simulink model "afe_abc_inv_psm_n"  (R2025b)
settings: Solver=ode1  StartTime=0.0  StopTime=simlength  FixedStep=tc  MaxStep=tc
values from neighbouring files (symbols this model uses):
  Adrso = eye(2) + Arso*ts_afe    [init_model.m]
  afe_pwm_phase_shift_mod1 = 0    [init_model.m]
  afe_pwm_phase_shift_mod2 = 0    [init_model.m]
  Aresd = eye(2) + Ares*ts_afe    [init_model.m]
  Bresd = Bres*ts_afe    [init_model.m]
  Cresd = Cres    [init_model.m]
  Crso = [1 0]    [init_model.m]
  CTRPIFF_CLIP_RELEASE = 0.001    [init_model.m]
  deepNEGeta = 0.5    [init_model.m]
  deepNEGxi = 0    [init_model.m]
  deepPOSxi = 0.5    [init_model.m]
  emf_fb_p = 0.2    [init_model.m]
  emf_fb_p_ccaller_1 = emf_fb_p    (= 0.2)    [init_model.m]
  emf_fb_p_ccaller_2 = emf_fb_p    (= 0.2)    [init_model.m]
  emf_p = emf_fb_p*4/10    (= 0.08)    [init_model.m]
  emf_p_ccaller_1 = emf_fb_p_ccaller_1*4/10    (= 0.08)    [init_model.m]
  emf_p_ccaller_2 = emf_fb_p_ccaller_2*4/10    (= 0.08)    [init_model.m]
  g0_161Hz = fcut_161Hz_flt * ts_afe * 2*pi    (= 0.126449104307)    [init_model.m]
  g0_1Hz = fcut_1Hz_flt * ts_afe * 2*pi    (= 0.000785398163397)    [init_model.m]
  g0_500Hz = fcut_500Hz_flt * ts_afe * 2*pi    (= 0.392699081699)    [init_model.m]
  g1_161Hz = 1 - g0_161Hz    (= 0.873550895693)    [init_model.m]
  g1_1Hz = 1 - g0_1Hz    (= 0.999214601837)    [init_model.m]
  g1_500Hz = 1 - g0_500Hz    (= 0.607300918301)    [init_model.m]
  i_grid_neg_eta_lim = 0.5    [init_model.m]
  i_grid_neg_eta_red_lim = 0.1    [init_model.m]
  i_grid_neg_xi_lim = 0.5    [init_model.m]
  i_grid_neg_xi_red_lim = 0.1    [init_model.m]
  i_grid_pos_eta_lim = 1    [init_model.m]
  i_grid_pos_eta_red_lim = 0.1    [init_model.m]
  id_lim = 0.35    [init_model.m]
  ieta_neg_ref_lim = 0.5    [init_model.m]
  ieta_pos_ref_lim = 1.0    (= 1)    [init_model.m]
  Igrid_phase_normalization_factor = 250e3/Vphase2/3/0.9*sqrt(2)    [init_model.m]
  inv_pwm_phase_shift_mod1 = 0    [init_model.m]
  iq_lim = 1.4    [init_model.m]
  ixi_pos_ref_lim = 1.6    [init_model.m]
  k_frt_ref = 2    [init_model.m]
  kg = Kobs(1)    [init_model.m]
  ki_afe = 45    [init_model.m]
  ki_align = 0.1    [init_model.m]
  ki_i = 18    [init_model.m]
  ki_rc_neg_grid = ki_rc_grid    (= 35)    [init_model.m]
  ki_rc_pos_grid = ki_rc_grid    (= 35)    [init_model.m]
  ki_vs = 35    [init_model.m]
  ki_w = 18    [init_model.m]
  kp_afe = 0.25    [init_model.m]
  kp_align = 0.6    [init_model.m]
  kp_i = 0.25    [init_model.m]
  kp_rc_neg_grid = kp_rc_grid    (= 0.35)    [init_model.m]
  kp_rc_pos_grid = kp_rc_grid    (= 0.35)    [init_model.m]
  kp_vs = 0.85    [init_model.m]
  kp_w = 2.5    [init_model.m]
  kw = Kobs(2)    [init_model.m]
  l1 = Kd(2)    [init_model.m]
  l2 = Kd(1)    [init_model.m]
  Ldrso = acker(Adrso',Crso',polesdrso)'    [init_model.m]
  lim_down_align = -0.2    [init_model.m]
  lim_up_align = 0.2    [init_model.m]
  mavarage_filter_frequency_base_order = 2    [init_model.m]
  motorc_m_scale = 2/3*Vdc_bez/ubez    [init_model.m]
  n1 = rms_perios/f_grid/ts_afe    [init_model.m]
  n10 = rms_perios/f_grid/ts_afe    [init_model.m]
  number_of_modules = 2    [init_model.m]
  omega_m_sim = omega_m_bez    [init_model.m]
  pll_i1 = 80    [init_model.m]
  pll_i1_ddsrt = pll_i1/2    (= 40)    [init_model.m]
  pll_p = 1    [init_model.m]
  pll_p_ddsrt = pll_p/2    (= 0.5)    [init_model.m]
  pll_p_frt = 0.2    [init_model.m]
  settle_time = 0.15    [init_model.m]
  simlength = 2    [init_model.m]
  start_time_LVRT = 2.0    (= 2)    [init_model.m]
  tc = ts_afe/200    (= 6.25e-07)    [init_model.m]
  time_aux_power_supply_fault = 1e3    (= 1000)    [init_model.m]
  time_gain_afe_module_1 = 1.0    (= 1)    [init_model.m]
  time_gain_afe_module_2 = 1.0    (= 1)    [init_model.m]
  time_gain_inv_module_1 = 1.0    (= 1)    [init_model.m]
  time_gain_inv_module_2 = 1.0    (= 1)    [init_model.m]
  time_phase_fault = 1e3    (= 1000)    [init_model.m]
  time_start_motor_control = 0.035    [init_model.m]
  transmission_delay = 125e-6*2    (= 0.00025)    [init_model.m]
  ts_afe = 1/fPWM_AFE/2    (= 0.000125)    [init_model.m]
  ts_inv = 1/fPWM_INV/2    (= 0.000125)    [init_model.m]
  Vdc_norm_ref = Vdc_ref/Vdc_nom    [init_model.m]
  Vdc_ref = 1070    [init_model.m]
  Vgrid_phase_normalization_factor = Vphase2*sqrt(2)    [init_model.m]
undefined symbols (not defined in the file or in its folder): Amplitude_U, Amplitude_V, Amplitude_W, end_time_LVRT, ibez, La, Lb, Ld_norm, Lq_norm, Ls_norm, magnitude, omega_bez, omega_grid_emulator_nom, omega_grid_nom, omega_m_bez, Phase_shift, psi_bez, psi_m, psi_m_norm, rpm_base, rpm_bez, Rs, Rs_norm, t_ramp, tau_bez, torque_base, ubez, ugrid_factor, V_phase_normalization_factor, Vdc_bez, Vemu_ref_norm, vn_eta_pu, vn_xi_pu, vp_xi_pu
libraries: fl_lib x215, nesl_utility x107, moving_average_filter x20, cstblocks x20, moving_average_filter_cc x16, simulink x6, threephase_inductor_lib x4, three_phase_pwm_modulator x4, single_phase_transformer_lib x3, power_meter_iec x1, flexshaft_lib x1, psm x1
(part 4 of 15)

== system afe_abc_inv_psm_n/afe_abc_inv_psm_mod1/afe/switch_2 ==
  Diode : fl_lib/Electrical/Electrical Elements/Diode  Vf=Vgamma V  Ron=Ron Ohm  Goff=1e-8 1/Ohm  i_specify=off  i_priority=None  i=0 A  i_nominal_specify=off  i_nominal_value=1  i_nominal_unit=A  v_specify=off  v_priority=None  v=0 V  v_nominal_specify=off  v_nominal_value=1  v_nominal_unit=V
  Switch : fl_lib/Electrical/Electrical Elements/Switch  R_closed=Ron Ohm  G_open=1e-8 1/Ohm  Threshold=7.5  i_specify=off  i_priority=None  i=0 A  i_nominal_specify=off  i_nominal_value=1  i_nominal_unit=A  v_specify=off  v_priority=None  v=0 V  v_nominal_specify=off  v_nominal_value=1  v_nominal_unit=V
  snubber : fl_lib/Electrical/Electrical Elements/Capacitor  c=Csnubber F  r=Rsnubber Ohm  g=0 1/Ohm  i_specify=off  i_priority=None  i=0 A  i_nominal_specify=off  i_nominal_value=1  i_nominal_unit=A  v_specify=off  v_priority=None  v=0 V  v_nominal_specify=off  v_nominal_value=1  v_nominal_unit=V  vc_specify=off  vc_priority=High  vc=0 V  vc_nominal_specify=off  vc_nominal_value=1  vc_nominal_unit=V
  G : PMIOPort  Side=Left
  C : PMIOPort  Port=2  Side=Left
  E : PMIOPort  Port=3  Side=Right
  connections:
  Switch/RConn2 -- C/RConn1 -- snubber/LConn1 -- Diode/RConn1
  Switch/RConn1 -- G/RConn1
  Switch/LConn1 -- E/RConn1 -- snubber/RConn1 -- Diode/LConn1

== system afe_abc_inv_psm_n/afe_abc_inv_psm_mod1/afe/switch_3 ==
  Diode : fl_lib/Electrical/Electrical Elements/Diode  Vf=Vgamma V  Ron=Ron Ohm  Goff=1e-8 1/Ohm  i_specify=off  i_priority=None  i=0 A  i_nominal_specify=off  i_nominal_value=1  i_nominal_unit=A  v_specify=off  v_priority=None  v=0 V  v_nominal_specify=off  v_nominal_value=1  v_nominal_unit=V
  Switch : fl_lib/Electrical/Electrical Elements/Switch  R_closed=Ron Ohm  G_open=1e-8 1/Ohm  Threshold=7.5  i_specify=off  i_priority=None  i=0 A  i_nominal_specify=off  i_nominal_value=1  i_nominal_unit=A  v_specify=off  v_priority=None  v=0 V  v_nominal_specify=off  v_nominal_value=1  v_nominal_unit=V
  snubber : fl_lib/Electrical/Electrical Elements/Capacitor  c=Csnubber F  r=Rsnubber Ohm  g=0 1/Ohm  i_specify=off  i_priority=None  i=0 A  i_nominal_specify=off  i_nominal_value=1  i_nominal_unit=A  v_specify=off  v_priority=None  v=0 V  v_nominal_specify=off  v_nominal_value=1  v_nominal_unit=V  vc_specify=off  vc_priority=High  vc=0 V  vc_nominal_specify=off  vc_nominal_value=1  vc_nominal_unit=V
  G : PMIOPort  Side=Left
  C : PMIOPort  Port=2  Side=Left
  E : PMIOPort  Port=3  Side=Right
  connections:
  Switch/RConn2 -- C/RConn1 -- snubber/LConn1 -- Diode/RConn1
  Switch/RConn1 -- G/RConn1
  Switch/LConn1 -- E/RConn1 -- snubber/RConn1 -- Diode/LConn1

== system afe_abc_inv_psm_n/afe_abc_inv_psm_mod1/afe/switch_4 ==
  Diode : fl_lib/Electrical/Electrical Elements/Diode  Vf=Vgamma V  Ron=Ron Ohm  Goff=1e-8 1/Ohm  i_specify=off  i_priority=None  i=0 A  i_nominal_specify=off  i_nominal_value=1  i_nominal_unit=A  v_specify=off  v_priority=None  v=0 V  v_nominal_specify=off  v_nominal_value=1  v_nominal_unit=V
  Switch : fl_lib/Electrical/Electrical Elements/Switch  R_closed=Ron Ohm  G_open=1e-8 1/Ohm  Threshold=7.5  i_specify=off  i_priority=None  i=0 A  i_nominal_specify=off  i_nominal_value=1  i_nominal_unit=A  v_specify=off  v_priority=None  v=0 V  v_nominal_specify=off  v_nominal_value=1  v_nominal_unit=V
  snubber : fl_lib/Electrical/Electrical Elements/Capacitor  c=Csnubber F  r=Rsnubber Ohm  g=0 1/Ohm  i_specify=off  i_priority=None  i=0 A  i_nominal_specify=off  i_nominal_value=1  i_nominal_unit=A  v_specify=off  v_priority=None  v=0 V  v_nominal_specify=off  v_nominal_value=1  v_nominal_unit=V  vc_specify=off  vc_priority=High  vc=0 V  vc_nominal_specify=off  vc_nominal_value=1  vc_nominal_unit=V
  G : PMIOPort  Side=Left
  C : PMIOPort  Port=2  Side=Left
  E : PMIOPort  Port=3  Side=Right
  connections:
  E/RConn1 -- Switch/LConn1 -- snubber/RConn1 -- Diode/LConn1
  Switch/RConn1 -- G/RConn1
  C/RConn1 -- Switch/RConn2 -- snubber/LConn1 -- Diode/RConn1

== system afe_abc_inv_psm_n/afe_abc_inv_psm_mod1/afe/switch_5 ==
  Diode : fl_lib/Electrical/Electrical Elements/Diode  Vf=Vgamma V  Ron=Ron Ohm  Goff=1e-8 1/Ohm  i_specify=off  i_priority=None  i=0 A  i_nominal_specify=off  i_nominal_value=1  i_nominal_unit=A  v_specify=off  v_priority=None  v=0 V  v_nominal_specify=off  v_nominal_value=1  v_nominal_unit=V
  Switch : fl_lib/Electrical/Electrical Elements/Switch  R_closed=Ron Ohm  G_open=1e-8 1/Ohm  Threshold=7.5  i_specify=off  i_priority=None  i=0 A  i_nominal_specify=off  i_nominal_value=1  i_nominal_unit=A  v_specify=off  v_priority=None  v=0 V  v_nominal_specify=off  v_nominal_value=1  v_nominal_unit=V
  snubber : fl_lib/Electrical/Electrical Elements/Capacitor  c=Csnubber F  r=Rsnubber Ohm  g=0 1/Ohm  i_specify=off  i_priority=None  i=0 A  i_nominal_specify=off  i_nominal_value=1  i_nominal_unit=A  v_specify=off  v_priority=None  v=0 V  v_nominal_specify=off  v_nominal_value=1  v_nominal_unit=V  vc_specify=off  vc_priority=High  vc=0 V  vc_nominal_specify=off  vc_nominal_value=1  vc_nominal_unit=V
  G : PMIOPort  Side=Left
  C : PMIOPort  Port=2  Side=Left
  E : PMIOPort  Port=3  Side=Right
  connections:
  Switch/RConn2 -- C/RConn1 -- snubber/LConn1 -- Diode/RConn1
  Switch/RConn1 -- G/RConn1
  Switch/LConn1 -- E/RConn1 -- snubber/RConn1 -- Diode/LConn1

== system afe_abc_inv_psm_n/afe_abc_inv_psm_mod1/afe/switch_6 ==
  Diode : fl_lib/Electrical/Electrical Elements/Diode  Vf=Vgamma V  Ron=Ron Ohm  Goff=1e-8 1/Ohm  i_specify=off  i_priority=None  i=0 A  i_nominal_specify=off  i_nominal_value=1  i_nominal_unit=A  v_specify=off  v_priority=None  v=0 V  v_nominal_specify=off  v_nominal_value=1  v_nominal_unit=V
  Switch : fl_lib/Electrical/Electrical Elements/Switch  R_closed=Ron Ohm  G_open=1e-8 1/Ohm  Threshold=7.5  i_specify=off  i_priority=None  i=0 A  i_nominal_specify=off  i_nominal_value=1  i_nominal_unit=A  v_specify=off  v_priority=None  v=0 V  v_nominal_specify=off  v_nominal_value=1  v_nominal_unit=V
  snubber : fl_lib/Electrical/Electrical Elements/Capacitor  c=Csnubber F  r=Rsnubber Ohm  g=0 1/Ohm  i_specify=off  i_priority=None  i=0 A  i_nominal_specify=off  i_nominal_value=1  i_nominal_unit=A  v_specify=off  v_priority=None  v=0 V  v_nominal_specify=off  v_nominal_value=1  v_nominal_unit=V  vc_specify=off  vc_priority=High  vc=0 V  vc_nominal_specify=off  vc_nominal_value=1  vc_nominal_unit=V
  G : PMIOPort  Side=Left
  C : PMIOPort  Port=2  Side=Left
  E : PMIOPort  Port=3  Side=Right
  connections:
  E/RConn1 -- Switch/LConn1 -- snubber/RConn1 -- Diode/LConn1
  Switch/RConn1 -- G/RConn1
  C/RConn1 -- Switch/RConn2 -- snubber/LConn1 -- Diode/RConn1

== system afe_abc_inv_psm_n/afe_abc_inv_psm_mod1/brake/switch_5 ==
  Diode : fl_lib/Electrical/Electrical Elements/Diode  Vf=Vgamma V  Ron=Ron Ohm  Goff=1e-8 1/Ohm  i_specify=off  i_priority=None  i=0 A  i_nominal_specify=off  i_nominal_value=1  i_nominal_unit=A  v_specify=off  v_priority=None  v=0 V  v_nominal_specify=off  v_nominal_value=1  v_nominal_unit=V
  Switch : fl_lib/Electrical/Electrical Elements/Switch  R_closed=Ron Ohm  G_open=1e-8 1/Ohm  Threshold=7.5  i_specify=off  i_priority=None  i=0 A  i_nominal_specify=off  i_nominal_value=1  i_nominal_unit=A  v_specify=off  v_priority=None  v=0 V  v_nominal_specify=off  v_nominal_value=1  v_nominal_unit=V
  G : PMIOPort  Side=Left
  C : PMIOPort  Port=2  Side=Left
  E : PMIOPort  Port=3  Side=Right
  connections:
  Switch/RConn2 -- C/RConn1 -- Diode/RConn1
  Switch/RConn1 -- G/RConn1
  Switch/LConn1 -- E/RConn1 -- Diode/LConn1

== system afe_abc_inv_psm_n/afe_abc_inv_psm_mod1/brake/switch_6 ==
  Diode : fl_lib/Electrical/Electrical Elements/Diode  Vf=Vgamma V  Ron=Ron Ohm  Goff=1e-8 1/Ohm  i_specify=off  i_priority=None  i=0 A  i_nominal_specify=off  i_nominal_value=1  i_nominal_unit=A  v_specify=off  v_priority=None  v=0 V  v_nominal_specify=off  v_nominal_value=1  v_nominal_unit=V
  C : PMIOPort  Side=Left
  E : PMIOPort  Port=2  Side=Right
  connections:
  E/RConn1 -- Diode/LConn1
  C/RConn1 -- Diode/RConn1

== system afe_abc_inv_psm_n/afe_abc_inv_psm_mod1/inverter/inverter ==
  duties_uvw : Inport
  Bus Selector : BusSelector  OutputSignals=gate_cmd_Q1,gate_cmd_Q2,gate_cmd_Q3,gate_cmd_Q4,gate_cmd_Q5,gate_cmd_Q6
  Current Sensor1 : fl_lib/Electrical/Electrical Sensors/Current Sensor
  Product{,1..5} (6 alike) : Product
  Simulink-PS Converter{,1..5} (6 alike) : nesl_utility/Simulink-PS Converter  PhysicalDomain=network_engine_domain  SubClassName=ps_input  LeftPortType=input  RightPortType=output  PseudoPeriodic=off  Frequencies=[]  NoiseDistribution=none  NoiseParameters=[]  Unit=1  AffineConversion=on  FilteringAndDerivatives=provide  SimscapeFilterOrder=1  InputFilterTimeConstant=0.001  UdotUserProvided=0
  Step : Step  Time=time_aux_power_supply_fault  Before=1  After=0  SampleTime=0
  ileg_dc_inv : nesl_utility/PS-Simulink Converter  PhysicalDomain=network_engine_domain  SubClassName=ps_output  LeftPortType=input  RightPortType=output  PseudoPeriodic=off  Frequencies=[]  VectorFormat=1-D array  Unit=A  AffineConversion=on
  sv_pwm : Subsystem
  switch_1 : Subsystem
      settings: PortSchema="{\"entries\":[{\"content\":{\"sides\":[{\"content\":{\"connectorIds\":[\"LConn1\"]},\"type\":\"ConnectorPlacement.EquallySpacedRectSide\",\"uuid\":\"9277da8d-d460-43e6-8478-dd662f15d226\"},{\"content\":{\"connectorIds\":[],\"side\":\"RIGHT\"},\"type\":\"ConnectorPlacement.EquallySpacedRectSide\",\"uuid\":\"a7ece396-f1d9-4f4f-a05b-db1fc65d6e1d\"},{\"content\":{\"connectorIds\":[\"LConn2\"],\"side\":\"TOP\"},\"type\":\"ConnectorPlacement.EquallySpacedRectSide\",\"uuid\":\"fdd70777-e9cf-4317-afb6-cae87f75d5b0\"},{\"content\":{\"connectorIds\":[\"RConn1\"],\"side\":\"BOTTOM\"},\"type\":\"ConnectorPlacement.EquallySpacedRectSide\",\"uuid\":\"2353ed68-b1a1-4775-9ca9-31e268d5443b\"}]},\"type\":\"ConnectorPlacement.EquallySpacedConnector\",\"uuid\":\"d5479f4c-4e65-4791-adcb-73df11f88590\"}],\"packageUris\":[\"http://schema.mathworks.com/mf0/Connector/R2020b\"],\"version\":\"1.0\"}"
  switch_2 : Subsystem
      settings: PortSchema="{\"entries\":[{\"content\":{\"sides\":[{\"content\":{\"connectorIds\":[\"LConn1\"]},\"type\":\"ConnectorPlacement.EquallySpacedRectSide\",\"uuid\":\"9277da8d-d460-43e6-8478-dd662f15d226\"},{\"content\":{\"connectorIds\":[],\"side\":\"RIGHT\"},\"type\":\"ConnectorPlacement.EquallySpacedRectSide\",\"uuid\":\"a7ece396-f1d9-4f4f-a05b-db1fc65d6e1d\"},{\"content\":{\"connectorIds\":[\"LConn2\"],\"side\":\"TOP\"},\"type\":\"ConnectorPlacement.EquallySpacedRectSide\",\"uuid\":\"fdd70777-e9cf-4317-afb6-cae87f75d5b0\"},{\"content\":{\"connectorIds\":[\"RConn1\"],\"side\":\"BOTTOM\"},\"type\":\"ConnectorPlacement.EquallySpacedRectSide\",\"uuid\":\"2353ed68-b1a1-4775-9ca9-31e268d5443b\"}]},\"type\":\"ConnectorPlacement.EquallySpacedConnector\",\"uuid\":\"d5479f4c-4e65-4791-adcb-73df11f88590\"}],\"packageUris\":[\"http://schema.mathworks.com/mf0/Connector/R2020b\"],\"version\":\"1.0\"}"
  switch_3 : Subsystem
      settings: PortSchema="{\"entries\":[{\"content\":{\"sides\":[{\"content\":{\"connectorIds\":[\"LConn1\"]},\"type\":\"ConnectorPlacement.EquallySpacedRectSide\",\"uuid\":\"9277da8d-d460-43e6-8478-dd662f15d226\"},{\"content\":{\"connectorIds\":[],\"side\":\"RIGHT\"},\"type\":\"ConnectorPlacement.EquallySpacedRectSide\",\"uuid\":\"a7ece396-f1d9-4f4f-a05b-db1fc65d6e1d\"},{\"content\":{\"connectorIds\":[\"LConn2\"],\"side\":\"TOP\"},\"type\":\"ConnectorPlacement.EquallySpacedRectSide\",\"uuid\":\"fdd70777-e9cf-4317-afb6-cae87f75d5b0\"},{\"content\":{\"connectorIds\":[\"RConn1\"],\"side\":\"BOTTOM\"},\"type\":\"ConnectorPlacement.EquallySpacedRectSide\",\"uuid\":\"2353ed68-b1a1-4775-9ca9-31e268d5443b\"}]},\"type\":\"ConnectorPlacement.EquallySpacedConnector\",\"uuid\":\"d5479f4c-4e65-4791-adcb-73df11f88590\"}],\"packageUris\":[\"http://schema.mathworks.com/mf0/Connector/R2020b\"],\"version\":\"1.0\"}"
  switch_4 : Subsystem
      settings: PortSchema="{\"entries\":[{\"content\":{\"sides\":[{\"content\":{\"connectorIds\":[\"LConn1\"]},\"type\":\"ConnectorPlacement.EquallySpacedRectSide\",\"uuid\":\"9277da8d-d460-43e6-8478-dd662f15d226\"},{\"content\":{\"connectorIds\":[],\"side\":\"RIGHT\"},\"type\":\"ConnectorPlacement.EquallySpacedRectSide\",\"uuid\":\"a7ece396-f1d9-4f4f-a05b-db1fc65d6e1d\"},{\"content\":{\"connectorIds\":[\"LConn2\"],\"side\":\"TOP\"},\"type\":\"ConnectorPlacement.EquallySpacedRectSide\",\"uuid\":\"fdd70777-e9cf-4317-afb6-cae87f75d5b0\"},{\"content\":{\"connectorIds\":[\"RConn1\"],\"side\":\"BOTTOM\"},\"type\":\"ConnectorPlacement.EquallySpacedRectSide\",\"uuid\":\"2353ed68-b1a1-4775-9ca9-31e268d5443b\"}]},\"type\":\"ConnectorPlacement.EquallySpacedConnector\",\"uuid\":\"d5479f4c-4e65-4791-adcb-73df11f88590\"}],\"packageUris\":[\"http://schema.mathworks.com/mf0/Connector/R2020b\"],\"version\":\"1.0\"}"
  switch_5 : Subsystem
      settings: PortSchema="{\"entries\":[{\"content\":{\"sides\":[{\"content\":{\"connectorIds\":[\"LConn1\"]},\"type\":\"ConnectorPlacement.EquallySpacedRectSide\",\"uuid\":\"9277da8d-d460-43e6-8478-dd662f15d226\"},{\"content\":{\"connectorIds\":[],\"side\":\"RIGHT\"},\"type\":\"ConnectorPlacement.EquallySpacedRectSide\",\"uuid\":\"a7ece396-f1d9-4f4f-a05b-db1fc65d6e1d\"},{\"content\":{\"connectorIds\":[\"LConn2\"],\"side\":\"TOP\"},\"type\":\"ConnectorPlacement.EquallySpacedRectSide\",\"uuid\":\"fdd70777-e9cf-4317-afb6-cae87f75d5b0\"},{\"content\":{\"connectorIds\":[\"RConn1\"],\"side\":\"BOTTOM\"},\"type\":\"ConnectorPlacement.EquallySpacedRectSide\",\"uuid\":\"2353ed68-b1a1-4775-9ca9-31e268d5443b\"}]},\"type\":\"ConnectorPlacement.EquallySpacedConnector\",\"uuid\":\"d5479f4c-4e65-4791-adcb-73df11f88590\"}],\"packageUris\":[\"http://schema.mathworks.com/mf0/Connector/R2020b\"],\"version\":\"1.0\"}"
  switch_6 : Subsystem
      settings: PortSchema="{\"entries\":[{\"content\":{\"sides\":[{\"content\":{\"connectorIds\":[\"LConn1\"]},\"type\":\"ConnectorPlacement.EquallySpacedRectSide\",\"uuid\":\"9277da8d-d460-43e6-8478-dd662f15d226\"},{\"content\":{\"connectorIds\":[],\"side\":\"RIGHT\"},\"type\":\"ConnectorPlacement.EquallySpacedRectSide\",\"uuid\":\"a7ece396-f1d9-4f4f-a05b-db1fc65d6e1d\"},{\"content\":{\"connectorIds\":[\"LConn2\"],\"side\":\"TOP\"},\"type\":\"ConnectorPlacement.EquallySpacedRectSide\",\"uuid\":\"fdd70777-e9cf-4317-afb6-cae87f75d5b0\"},{\"content\":{\"connectorIds\":[\"RConn1\"],\"side\":\"BOTTOM\"},\"type\":\"ConnectorPlacement.EquallySpacedRectSide\",\"uuid\":\"2353ed68-b1a1-4775-9ca9-31e268d5443b\"}]},\"type\":\"ConnectorPlacement.EquallySpacedConnector\",\"uuid\":\"d5479f4c-4e65-4791-adcb-73df11f88590\"}],\"packageUris\":[\"http://schema.mathworks.com/mf0/Connector/R2020b\"],\"version\":\"1.0\"}"
  u : PMIOPort  Side=Left
  v : PMIOPort  Port=2  Side=Left
  w : PMIOPort  Port=3  Side=Left
  V+ : PMIOPort  Port=4  Side=Right
  V- : PMIOPort  Port=5  Side=Right
  tag scope: ileg_dc_inv_mod1=global
  wires:
  [I1] -> Simulink-PS Converter/1
  [I2] -> Simulink-PS Converter1/1
  [I3] -> Simulink-PS Converter2/1
  [I4] -> Simulink-PS Converter3/1
  [I5] -> Simulink-PS Converter4/1
  [I6] -> Simulink-PS Converter5/1
  sv_pwm/1(gate_cmds) -> Bus Selector/1
  ileg_dc_inv/1 -> [ileg_dc_inv_mod1]
  Product/1 -> [I1]
  Product3/1 -> [I4]
  Product4/1 -> [I5]
  Product5/1 -> [I6]
  Product2/1 -> [I3]
  Product1/1 -> [I2]
  Step/1 -> Product5/1, Product4/1, Product3/1, Product2/1, Product/1, Product1/1
  Bus Selector/1 -> Product/2  "<gate_cmd_Q1>"
  Bus Selector/2 -> Product1/2  "<gate_cmd_Q2>"
  Bus Selector/3 -> Product2/2  "<gate_cmd_Q3>"
  Bus Selector/4 -> Product3/2  "<gate_cmd_Q4>"
  Bus Selector/5 -> Product4/2  "<gate_cmd_Q5>"
  Bus Selector/6 -> Product5/2  "<gate_cmd_Q6>"
  duties_uvw/1 -> sv_pwm/1(duties_uvw)
  connections:
  Current Sensor1/LConn1 -- V+/RConn1 -- switch_5/LConn2 -- switch_3/LConn2
  V-/RConn1 -- switch_2/RConn1 -- switch_6/RConn1 -- switch_4/RConn1
  switch_1/LConn1 -- Simulink-PS Converter/RConn1
  switch_2/LConn1 -- Simulink-PS Converter1/RConn1
  switch_3/LConn1 -- Simulink-PS Converter2/RConn1
  switch_4/LConn1 -- Simulink-PS Converter3/RConn1
  switch_5/LConn1 -- Simulink-PS Converter4/RConn1
  switch_6/LConn1 -- Simulink-PS Converter5/RConn1
  u/RConn1 -- switch_2/LConn2 -- switch_1/RConn1
  v/RConn1 -- switch_4/LConn2 -- switch_3/RConn1
  w/RConn1 -- switch_6/LConn2 -- switch_5/RConn1
  switch_1/LConn2 -- Current Sensor1/RConn2
  Current Sensor1/RConn1 -- ileg_dc_inv/LConn1

== system afe_abc_inv_psm_n/afe_abc_inv_psm_mod2/AFE_control/afe_control ==
  ug_abc_pu : Inport
  udc_pu : Inport  Port=2
  ig_abc_pu : Inport  Port=3
  is_abc_pu : Inport  Port=4
  local_time : Inport  Port=5
  master_time : Inport  Port=6
  Trigger : TriggerPort  VariantControl=(inherit)  PortDimensions=1
  Constant : Constant  Value=Vdc_norm_ref
  FRT-VDE4110 : Subsystem
  To Workspace4 : ToWorkspace  VariableName=t_ts_afe_sim_mod2  SampleTime=-1
      settings: MaxDataPoints=Ns_afe
  current_ctrl : Subsystem
  data_to_worspace_module_1 : Subsystem
  grid_current_sequences_and_reactive_pwr_ctrl : Subsystem
  grid_voltage_phase_lock_loops : Subsystem
  grid_voltage_sequences : Subsystem
  ig afe quantizzation and one step delay : Subsystem
  instantaneus_power : Subsystem
  interesting scopes : Subsystem
  is afe quantizzation and one step delay : Subsystem
  islanding_mode_detector : Subsystem
  phase_compensation_1 : Subsystem
  power-meter mod1 : Scope  NumInputPorts=2
      settings: ActiveDisplayYMinimum=-41.328407089198727  ActiveDisplayYMaximum=23.571293495272425  DataLoggingVariableName=ScopeData9
  space_vector : Subsystem
  udc_acquisition : Subsystem
  udc_ctrl : Subsystem
  ug afe quantizzation and one step delay : Subsystem
  duvw : Outport
  AFE2_local_time_corr : Outport  Port=2
  tag scope: igd_abc_pu_mod2=global, isd_abc_pu_mod2=global, udcd_pu_afe_mod2=global, ugd_abc_pu_mod2=global
  wires:
  [ug_beta_pu_mod2] -> islanding_mode_detector/3(beta)
  ig afe quantizzation and one step delay/1(igd_abc_pu) -> [igd_abc_pu_mod2]
  is afe quantizzation and one step delay/1(isd_abc_pu) -> [isd_abc_pu_mod2]
  ug afe quantizzation and one step delay/1(ugd_abc_pu) -> [ugd_abc_pu_mod2]
  [ug_alpha_pu_mod2] -> islanding_mode_detector/2(alpha)
  [gamma_grid_pll_mod2] -> islanding_mode_detector/1(gamma)
  [pwr_act_grid_mod2] -> power-meter mod1/1  "pwr_act_grid_mod1(kW)"
  [pwr_react_grid_mod2] -> power-meter mod1/2  "pwr_react_grid_mod1(kVAr)"
  udc_acquisition/1(udcd_pu) -> [udcd_pu_afe_mod2]
  udc_pu/1 -> udc_acquisition/1(udc_pu)
  [udcd_pu_afe_mod2] -> udc_ctrl/1(udc_pu)
  [isd_abc_pu_mod2] -> current_ctrl/2(is_abc_pu)
  [igd_abc_pu_mod2] -> grid_current_sequences_and_reactive_pwr_ctrl/1(ig_abc_pu)
  [ugd_abc_pu_mod2] -> grid_voltage_phase_lock_loops/1(ug_abc_pu)
  ig_abc_pu/1 -> ig afe quantizzation and one step delay/1(ig_abc_pu)
  is_abc_pu/1 -> is afe quantizzation and one step delay/1(is_abc_pu)
  space_vector/1(duvw) -> duvw/1
  current_ctrl/1(uab_out) -> space_vector/1(uab_out)
  ug_abc_pu/1 -> ug afe quantizzation and one step delay/1(ug_abc_pu)
  udc_ctrl/1(i_xi_ref) -> current_ctrl/1(i_xi_ref)  "i_xi_ref"
  Constant/1 -> udc_ctrl/2(udc_pu_ref)
  local_time/1 -> [local_time], To Workspace4/1
  [local_time] -> phase_compensation_1/1(local_time)
  phase_compensation_1/1(y) -> AFE2_local_time_corr/1
  master_time/1 -> phase_compensation_1/2(master_time)

== system afe_abc_inv_psm_n/afe_abc_inv_psm_mod2/INV_control/inverter_control ==
  is_uvw : Inport
  udc_pu : Inport  Port=2
  local_time : Inport  Port=3
  master_time : Inport  Port=4
  master_torque_ref : Inport  Port=5
  theta_elec_psm : Inport  Port=6
  Trigger : TriggerPort  VariantControl=(inherit)  PortDimensions=1
  Bus Creator : BusCreator  Inputs=2
  Mux2 : Mux  Inputs=3
  To Workspace1 : ToWorkspace  VariableName=t_ts_inv_sim_mod2  SampleTime=-1
      settings: MaxDataPoints=Ns_afe
  Variant Source : VariantSource  VariantControls={use_torque_curve == 1, use_speed_control == 1}
  current_ctrl : Subsystem
  encoder-sensorless-switch : Subsystem
  is inv quantizzation and one step delay : Subsystem
  measurements : Subsystem
  omega_pu : Subsystem
  omega_ref/omega_mod2 : Scope  NumInputPorts=3
      settings: ActiveDisplayYMinimum=-1.3333452178372498  ActiveDisplayYMaximum=1.261433879815884  DataLoggingVariableName=ScopeData3
  phase_compensation_1 : Subsystem
  space_vector : Subsystem
  torque_reference : Subsystem
  udc_acquisition : Subsystem
  duvw : Outport  VectorParamsAs1DForOutWhenUnconnected=off
  INV2_local_time_corr : Outport  Port=2
  tag scope: isd_uvw_inv_mod2=global, udcd_pu_inv_mod2=global
  wires:
  is inv quantizzation and one step delay/1(isd_abc_pu) -> [isd_uvw_inv_mod2]
  is_uvw/1 -> is inv quantizzation and one step delay/1(is_abc_pu)
  udc_pu/1 -> udc_acquisition/1(udc_pu)
  udc_acquisition/1(udcd_pu) -> [udcd_pu_inv_mod2]
  master_torque_ref/1 -> Variant Source/2, Bus Creator/2  "master_torque_ref"
  torque_reference/1(torque_ref) -> Variant Source/1  "iq_ref"
  omega_pu/1(abs(omega_pu)) -> torque_reference/1(rotor speed)
  omega_pu/2(omega_pu) -> Bus Creator/1  "omega_hat_pu"
  [u_mot_pu_mod2] -> Mux2/3  "u_mot_pu_mod2"
  Mux2/1 -> omega_ref/omega_mod2/3
  [uq_pu_mod2] -> Mux2/2  "uq_pu_mod2"
  [ud_pu_mod2] -> Mux2/1  "ud_pu_mod2"
  Variant Source/1 -> current_ctrl/1(torque_ref), omega_ref/omega_mod2/2  "torque reference"
  Bus Creator/1 -> omega_ref/omega_mod2/1  "x"
  local_time/1 -> To Workspace1/1, [local_time]
  phase_compensation_1/1(y) -> INV2_local_time_corr/1
  master_time/1 -> phase_compensation_1/2(master_time)
  [local_time] -> phase_compensation_1/1(local_time)
  current_ctrl/1(uab) -> space_vector/1(uab)
  space_vector/1(duvw) -> duvw/1
  theta_elec_psm/1 -> encoder-sensorless-switch/1(theta_elec_psm)

== system afe_abc_inv_psm_n/afe_abc_inv_psm_mod2/LCL_filter/threephase_vi_measures_stack ==
  Bus Creator : BusCreator  Inputs=6
  Current Sensor : fl_lib/Electrical/Electrical Sensors/Current Sensor
  Current Sensor1 : fl_lib/Electrical/Electrical Sensors/Current Sensor
  Current Sensor2 : fl_lib/Electrical/Electrical Sensors/Current Sensor
  Electrical Reference1 : fl_lib/Electrical/Electrical Elements/Electrical Reference
  Gain : Gain  Gain=1/3
  Gain1 : Gain  Gain=1/Vgrid_phase_normalization_factor
  Gain2 : Gain  Gain=1/Vgrid_phase_normalization_factor
  Gain3 : Gain  Gain=1/Vgrid_phase_normalization_factor
  Gain4 : Gain  Gain=1/Igrid_phase_normalization_factor
  Gain5 : Gain  Gain=1/Igrid_phase_normalization_factor
  Gain6 : Gain  Gain=1/Igrid_phase_normalization_factor
  Gain7 : Gain  Gain=Igrid_phase_normalization_factor
  Gain8 : Gain  Gain=Vgrid_phase_normalization_factor
  Gain9 : Gain  Gain=Igrid_phase_normalization_factor
  Selector : Selector  InputPortWidth=6  IndexOptions=Index vector (dialog)  Indices=[1 2 3]  OutputSizes=1
  Selector1 : Selector  InputPortWidth=6  IndexOptions=Index vector (dialog)  Indices=[4 5 6]  OutputSizes=1
  Sum : Sum  Inputs=+++
  Voltage Sensor : fl_lib/Electrical/Electrical Sensors/Voltage Sensor
  Voltage Sensor1 : fl_lib/Electrical/Electrical Sensors/Voltage Sensor
  Voltage Sensor2 : fl_lib/Electrical/Electrical Sensors/Voltage Sensor
  ia_afe : nesl_utility/PS-Simulink Converter  PhysicalDomain=network_engine_domain  SubClassName=ps_output  LeftPortType=input  RightPortType=output  PseudoPeriodic=off  Frequencies=[]  VectorFormat=1-D array  Unit=A  AffineConversion=off
  ib_afe : nesl_utility/PS-Simulink Converter  PhysicalDomain=network_engine_domain  SubClassName=ps_output  LeftPortType=input  RightPortType=output  PseudoPeriodic=off  Frequencies=[]  VectorFormat=1-D array  Unit=A  AffineConversion=off
  ic_afe : nesl_utility/PS-Simulink Converter  PhysicalDomain=network_engine_domain  SubClassName=ps_output  LeftPortType=input  RightPortType=output  PseudoPeriodic=off  Frequencies=[]  VectorFormat=1-D array  Unit=A  AffineConversion=off
  is_abc/us_abc _mod2 : Scope  NumInputPorts=3
      settings: SampleTime=tc  ActiveDisplayYMinimum=-383.27868862774517  ActiveDisplayYMaximum=384.39078927767747
  ua_afe : nesl_utility/PS-Simulink Converter  PhysicalDomain=network_engine_domain  SubClassName=ps_output  LeftPortType=input  RightPortType=output  PseudoPeriodic=off  Frequencies=[]  VectorFormat=1-D array  Unit=V  AffineConversion=off
  ub_afe : nesl_utility/PS-Simulink Converter  PhysicalDomain=network_engine_domain  SubClassName=ps_output  LeftPortType=input  RightPortType=output  PseudoPeriodic=off  Frequencies=[]  VectorFormat=1-D array  Unit=V  AffineConversion=off
  uc_afe : nesl_utility/PS-Simulink Converter  PhysicalDomain=network_engine_domain  SubClassName=ps_output  LeftPortType=input  RightPortType=output  PseudoPeriodic=off  Frequencies=[]  VectorFormat=1-D array  Unit=V  AffineConversion=off
  Ua : PMIOPort  Side=Left
  ua : PMIOPort  Port=2  Side=Right
  Ub : PMIOPort  Port=3  Side=Left
  ub : PMIOPort  Port=4  Side=Right
  Uc : PMIOPort  Port=5  Side=Left
  uc : PMIOPort  Port=6  Side=Right
  tag scope: is_abc_pu_mod2=global, iz_afe_pu_mod2=global, vs_abc_pu_mod2=global
  wires:
  Gain9/1 -> is_abc/us_abc _mod2/3  "iz_afe_mod2"
  Gain8/1 -> is_abc/us_abc _mod2/2  "vs_abc_mod2"
  Gain7/1 -> is_abc/us_abc _mod2/1  "is_abc_mod2"
  Gain5/1 -> Sum/3, Bus Creator/6  "ic_afe_pu"
  Gain4/1 -> Bus Creator/5, Sum/2  "ib_afe_pu"
  Gain6/1 -> Bus Creator/4, Sum/1  "ia_afe_pu"
  Gain3/1 -> Bus Creator/3  "uc_afe_pu"
  Gain2/1 -> Bus Creator/2  "ub_afe_pu"
  Gain1/1 -> Bus Creator/1  "ua_afe_pu"
  [iz_afe_pu_mod2] -> Gain9/1
  Gain/1 -> [iz_afe_pu_mod2]
  Sum/1 -> Gain/1
  [vs_abc_pu_mod2] -> Gain8/1
  [is_abc_pu_mod2] -> Gain7/1
  Selector1/1 -> [is_abc_pu_mod2]
  uc_afe/1 -> Gain3/1  "uc_afe"
  ub_afe/1 -> Gain2/1  "ub_afe"
  ua_afe/1 -> Gain1/1  "ua_afe"
  ic_afe/1 -> Gain5/1  "ic_afe"
  ia_afe/1 -> Gain6/1  "ia_afe"
  ib_afe/1 -> Gain4/1  "ib_afe"
  Selector/1 -> [vs_abc_pu_mod2]
  Bus Creator/1 -> Selector1/1, Selector/1  "vi_data"
  connections:
  Current Sensor2/RConn2 -- uc/RConn1
  ic_afe/LConn1 -- Current Sensor2/RConn1
  ia_afe/LConn1 -- Current Sensor/RConn1
  ib_afe/LConn1 -- Current Sensor1/RConn1
  Voltage Sensor2/RConn1 -- uc_afe/LConn1
  Current Sensor1/RConn2 -- ub/RConn1
  Voltage Sensor/LConn1 -- Ua/RConn1 -- Current Sensor/LConn1
  Current Sensor2/LConn1 -- Uc/RConn1 -- Voltage Sensor2/LConn1
  Voltage Sensor1/RConn1 -- ub_afe/LConn1
  Current Sensor/RConn2 -- ua/RConn1
  Voltage Sensor/RConn1 -- ua_afe/LConn1
  Voltage Sensor1/RConn2 -- Voltage Sensor2/RConn2 -- Voltage Sensor/RConn2 -- Electrical Reference1/LConn1
  Voltage Sensor1/LConn1 -- Ub/RConn1 -- Current Sensor1/LConn1

== system afe_abc_inv_psm_n/afe_abc_inv_psm_mod2/LCL_filter/threephase_vi_measures_stack1 ==
  Bus Creator : BusCreator  Inputs=6
  Current Sensor : fl_lib/Electrical/Electrical Sensors/Current Sensor
  Current Sensor1 : fl_lib/Electrical/Electrical Sensors/Current Sensor
  Current Sensor2 : fl_lib/Electrical/Electrical Sensors/Current Sensor
  Electrical Reference1 : fl_lib/Electrical/Electrical Elements/Electrical Reference
  Gain : Gain  Gain=1/Vgrid_phase_normalization_factor
  Gain1 : Gain  Gain=1/Vgrid_phase_normalization_factor
  Gain10 : Gain  Gain=1/Igrid_phase_normalization_factor
  Gain2 : Gain  Gain=1/Vgrid_phase_normalization_factor
  Gain6 : Gain  Gain=1/Igrid_phase_normalization_factor
  Gain9 : Gain  Gain=1/Igrid_phase_normalization_factor
  Selector : Selector  InputPortWidth=6  IndexOptions=Index vector (dialog)  Indices=[1 2 3]  OutputSizes=1
  Selector1 : Selector  InputPortWidth=6  IndexOptions=Index vector (dialog)  Indices=[4 5 6]  OutputSizes=1
  Voltage Sensor : fl_lib/Electrical/Electrical Sensors/Voltage Sensor
  Voltage Sensor1 : fl_lib/Electrical/Electrical Sensors/Voltage Sensor
  Voltage Sensor2 : fl_lib/Electrical/Electrical Sensors/Voltage Sensor
  ia_grid : nesl_utility/PS-Simulink Converter  PhysicalDomain=network_engine_domain  SubClassName=ps_output  LeftPortType=input  RightPortType=output  PseudoPeriodic=off  Frequencies=[]  VectorFormat=1-D array  Unit=A  AffineConversion=off
  ib_grid : nesl_utility/PS-Simulink Converter  PhysicalDomain=network_engine_domain  SubClassName=ps_output  LeftPortType=input  RightPortType=output  PseudoPeriodic=off  Frequencies=[]  VectorFormat=1-D array  Unit=A  AffineConversion=off
  ic_grid : nesl_utility/PS-Simulink Converter  PhysicalDomain=network_engine_domain  SubClassName=ps_output  LeftPortType=input  RightPortType=output  PseudoPeriodic=off  Frequencies=[]  VectorFormat=1-D array  Unit=A  AffineConversion=off
  ig_abc/ug_abc _mod2 : Scope  NumInputPorts=2
      settings: SampleTime=tc  ActiveDisplayYMinimum=-335.78711  ActiveDisplayYMaximum=237.87058
  ua_grid : nesl_utility/PS-Simulink Converter  PhysicalDomain=network_engine_domain  SubClassName=ps_output  LeftPortType=input  RightPortType=output  PseudoPeriodic=off  Frequencies=[]  VectorFormat=1-D array  Unit=V  AffineConversion=off
  ub_grid : nesl_utility/PS-Simulink Converter  PhysicalDomain=network_engine_domain  SubClassName=ps_output  LeftPortType=input  RightPortType=output  PseudoPeriodic=off  Frequencies=[]  VectorFormat=1-D array  Unit=V  AffineConversion=off
  uc_grid : nesl_utility/PS-Simulink Converter  PhysicalDomain=network_engine_domain  SubClassName=ps_output  LeftPortType=input  RightPortType=output  PseudoPeriodic=off  Frequencies=[]  VectorFormat=1-D array  Unit=V  AffineConversion=off
  Ua : PMIOPort  Side=Left
  ua : PMIOPort  Port=2  Side=Right
  Ub : PMIOPort  Port=3  Side=Left
  ub : PMIOPort  Port=4  Side=Right
  Uc : PMIOPort  Port=5  Side=Left
  uc : PMIOPort  Port=6  Side=Right
  tag scope: ig_abc_pu_mod2=global, ug_abc_pu_mod2=global
  wires:
  Gain10/1 -> Bus Creator/6  "ic_grid_pu"
  Gain9/1 -> Bus Creator/5  "ib_grid_pu"
  Gain6/1 -> Bus Creator/4  "ia_grid_pu"
  Gain2/1 -> Bus Creator/3  "uc_grid_pu"
  Gain1/1 -> Bus Creator/2  "ub_grid_pu"
  Gain/1 -> Bus Creator/1  "ua_grid_pu"
  Bus Creator/1 -> Selector1/1, Selector/1  "vi_data"
  Selector/1 -> [ug_abc_pu_mod2]
  ib_grid/1 -> Gain9/1
  ia_grid/1 -> Gain6/1
  ic_grid/1 -> Gain10/1
  ua_grid/1 -> Gain/1
  ub_grid/1 -> Gain1/1
  uc_grid/1 -> Gain2/1
  Selector1/1 -> [ig_abc_pu_mod2]
  [ig_abc_pu_mod2] -> ig_abc/ug_abc _mod2/1  "ig_abc_mod2"
  [ug_abc_pu_mod2] -> ig_abc/ug_abc _mod2/2  "ug_abc_mod2"
  connections:
  Current Sensor1/LConn1 -- Ub/RConn1 -- Voltage Sensor1/LConn1
  Electrical Reference1/LConn1 -- Voltage Sensor/RConn2 -- Voltage Sensor2/RConn2 -- Voltage Sensor1/RConn2
  Voltage Sensor/RConn1 -- ua_grid/LConn1
  Current Sensor/RConn2 -- ua/RConn1
  Voltage Sensor1/RConn1 -- ub_grid/LConn1
  Voltage Sensor2/LConn1 -- Uc/RConn1 -- Current Sensor2/LConn1
  Current Sensor/LConn1 -- Ua/RConn1 -- Voltage Sensor/LConn1
  Current Sensor1/RConn2 -- ub/RConn1
  Voltage Sensor2/RConn1 -- uc_grid/LConn1
  ib_grid/LConn1 -- Current Sensor1/RConn1
  ia_grid/LConn1 -- Current Sensor/RConn1
  ic_grid/LConn1 -- Current Sensor2/RConn1
  Current Sensor2/RConn2 -- uc/RConn1

== system afe_abc_inv_psm_n/afe_abc_inv_psm_mod2/L_filter/threephase_vi_measures_stack ==
  Bus Creator : BusCreator  Inputs=6
  Current Sensor : fl_lib/Electrical/Electrical Sensors/Current Sensor
  Current Sensor1 : fl_lib/Electrical/Electrical Sensors/Current Sensor
  Current Sensor2 : fl_lib/Electrical/Electrical Sensors/Current Sensor
  Electrical Reference1 : fl_lib/Electrical/Electrical Elements/Electrical Reference
  Gain : Gain  Gain=1/ibez
  Gain1 : Gain  Gain=1/ibez
  Gain2 : Gain  Gain=1/ibez
  Gain3 : Gain  Gain=1/ubez
  Gain4 : Gain  Gain=1/ubez
  Gain5 : Gain  Gain=1/ubez
  Selector : Selector  InputPortWidth=6  IndexOptions=Index vector (dialog)  Indices=[1 2 3]  OutputSizes=1
  Selector1 : Selector  InputPortWidth=6  IndexOptions=Index vector (dialog)  Indices=[4 5 6]  OutputSizes=1
  Voltage Sensor : fl_lib/Electrical/Electrical Sensors/Voltage Sensor
  Voltage Sensor1 : fl_lib/Electrical/Electrical Sensors/Voltage Sensor
  Voltage Sensor2 : fl_lib/Electrical/Electrical Sensors/Voltage Sensor
  iu_inv : nesl_utility/PS-Simulink Converter  PhysicalDomain=network_engine_domain  SubClassName=ps_output  LeftPortType=input  RightPortType=output  PseudoPeriodic=off  Frequencies=[]  VectorFormat=1-D array  Unit=A  AffineConversion=off
  iv_inv : nesl_utility/PS-Simulink Converter  PhysicalDomain=network_engine_domain  SubClassName=ps_output  LeftPortType=input  RightPortType=output  PseudoPeriodic=off  Frequencies=[]  VectorFormat=1-D array  Unit=A  AffineConversion=off
  iw_inv : nesl_utility/PS-Simulink Converter  PhysicalDomain=network_engine_domain  SubClassName=ps_output  LeftPortType=input  RightPortType=output  PseudoPeriodic=off  Frequencies=[]  VectorFormat=1-D array  Unit=A  AffineConversion=off
  uu_inv : nesl_utility/PS-Simulink Converter  PhysicalDomain=network_engine_domain  SubClassName=ps_output  LeftPortType=input  RightPortType=output  PseudoPeriodic=off  Frequencies=[]  VectorFormat=1-D array  Unit=V  AffineConversion=off
  uv_inv : nesl_utility/PS-Simulink Converter  PhysicalDomain=network_engine_domain  SubClassName=ps_output  LeftPortType=input  RightPortType=output  PseudoPeriodic=off  Frequencies=[]  VectorFormat=1-D array  Unit=V  AffineConversion=off
  uw_inv : nesl_utility/PS-Simulink Converter  PhysicalDomain=network_engine_domain  SubClassName=ps_output  LeftPortType=input  RightPortType=output  PseudoPeriodic=off  Frequencies=[]  VectorFormat=1-D array  Unit=V  AffineConversion=off
  Uu : PMIOPort  Side=Left
  uu : PMIOPort  Port=2  Side=Right
  Uv : PMIOPort  Port=3  Side=Left
  uv : PMIOPort  Port=4  Side=Right
  Uw : PMIOPort  Port=5  Side=Left
  uw : PMIOPort  Port=6  Side=Right
  tag scope: is_uvw_pu_mod2=global, us_uvw_pu_mod2=global
  wires:
  Gain5/1 -> Bus Creator/3  "uw_inv_pu"
  Gain4/1 -> Bus Creator/2  "uv_inv_pu"
  Gain3/1 -> Bus Creator/1  "uu_inv_pu"
  Gain2/1 -> Bus Creator/6  "iw_inv_pu"
  Gain1/1 -> Bus Creator/5  "iv_inv_pu"
  Gain/1 -> Bus Creator/4  "iu_inv_pu"
  Selector1/1 -> [is_uvw_pu_mod2]
  uw_inv/1 -> Gain5/1  "uw_inv"
  uv_inv/1 -> Gain4/1  "uv_inv"
  uu_inv/1 -> Gain3/1  "uu_inv"
  iw_inv/1 -> Gain2/1  "iw_inv"
  iu_inv/1 -> Gain/1  "iu_inv"
  iv_inv/1 -> Gain1/1  "iv_inv"
  Selector/1 -> [us_uvw_pu_mod2]
  Bus Creator/1 -> Selector1/1, Selector/1  "vi_data"
  connections:
  Current Sensor2/RConn2 -- uw/RConn1
  iw_inv/LConn1 -- Current Sensor2/RConn1
  iu_inv/LConn1 -- Current Sensor/RConn1
  iv_inv/LConn1 -- Current Sensor1/RConn1
  Voltage Sensor2/RConn1 -- uw_inv/LConn1
  Current Sensor1/RConn2 -- uv/RConn1
  Voltage Sensor/LConn1 -- Uu/RConn1 -- Current Sensor/LConn1
  Current Sensor2/LConn1 -- Uw/RConn1 -- Voltage Sensor2/LConn1
  Voltage Sensor1/RConn1 -- uv_inv/LConn1
  Current Sensor/RConn2 -- uu/RConn1
  Voltage Sensor/RConn1 -- uu_inv/LConn1
  Voltage Sensor1/RConn2 -- Voltage Sensor2/RConn2 -- Voltage Sensor/RConn2 -- Electrical Reference1/LConn1
  Voltage Sensor1/LConn1 -- Uv/RConn1 -- Current Sensor1/LConn1

== system afe_abc_inv_psm_n/afe_abc_inv_psm_mod2/afe/dclink_measure ==
  Controlled Voltage Source : fl_lib/Electrical/Electrical Sources/Controlled Voltage Source
  Current Sensor1 : fl_lib/Electrical/Electrical Sensors/Current Sensor
  Electrical Reference : fl_lib/Electrical/Electrical Elements/Electrical Reference
  Gain : Gain  Gain=107.4e3
  Gain1 : Gain  Gain=1/Vdc_bez
  R_derating : Subsystem  Commented=on
  Resistor : fl_lib/Electrical/Electrical Elements/Resistor  R=107.4 kOhm  i_specify=off  i_priority=None  i=0 A  i_nominal_specify=off  i_nominal_value=1  i_nominal_unit=A  v_specify=off  v_priority=None  v=0 V  v_nominal_specify=off  v_nominal_value=1  v_nominal_unit=V
  Saturation : Saturate  UpperLimit=inf  LowerLimit=1
  Simulink-PS Converter : nesl_utility/Simulink-PS Converter  PhysicalDomain=network_engine_domain  SubClassName=ps_input  LeftPortType=input  RightPortType=output  PseudoPeriodic=off  Frequencies=[]  NoiseDistribution=none  NoiseParameters=[]  Unit=Ohm  AffineConversion=off  FilteringAndDerivatives=provide  SimscapeFilterOrder=1  InputFilterTimeConstant=0.001  UdotUserProvided=0
  Variable Resistor : fl_lib/Electrical/Electrical Elements/Variable Resistor  Rmin=0 Ohm  thermalEnable=false  thermal_mass=1 J/K  i_specify=off  i_priority=None  i=0 A  i_nominal_specify=off  i_nominal_value=1  i_nominal_unit=A  v_specify=off  v_priority=None  v=0 V  v_nominal_specify=off  v_nominal_value=1  v_nominal_unit=V  T_specify=off  T_priority=None  T=300 K  T_nominal_specify=off  T_nominal_value=1  T_nominal_unit=K
  dclink_voltage_measure_comparison mod2 : Scope  NumInputPorts=3
      settings: SampleTime=tc  ActiveDisplayYMinimum=439.20035  ActiveDisplayYMaximum=1355.17542
  im_udc : nesl_utility/PS-Simulink Converter  PhysicalDomain=network_engine_domain  SubClassName=ps_output  LeftPortType=input  RightPortType=output  PseudoPeriodic=off  Frequencies=[]  VectorFormat=1-D array  Unit=A  AffineConversion=on
  udc : PMIOPort  Side=Left
  tag scope: vdc_pu_afe_mod2=global, vdc_pu_inv_mod2=global
  wires:
  Gain1/1 -> [vdc_pu_afe_mod2], dclink_voltage_measure_comparison mod2/2, [vdc_pu_inv_mod2]
  R_derating/1(DR) -> Simulink-PS Converter/1
  [udc_mod2] -> dclink_voltage_measure_comparison mod2/3  "real"
  im_udc/1 -> Gain/1
  Saturation/1 -> Gain1/1
  Gain/1 -> dclink_voltage_measure_comparison mod2/1, Saturation/1  "measure_si"
  connections:
  Controlled Voltage Source/LConn1 -- Resistor/LConn1
  Simulink-PS Converter/RConn1 -- Variable Resistor/LConn1
  Current Sensor1/LConn1 -- Variable Resistor/RConn1
  Controlled Voltage Source/RConn2 -- Electrical Reference/LConn1 -- Current Sensor1/RConn2
  Current Sensor1/RConn1 -- im_udc/LConn1
  Resistor/RConn1 -- Variable Resistor/LConn2
  udc/RConn1 -- Controlled Voltage Source/RConn1

== system afe_abc_inv_psm_n/afe_abc_inv_psm_mod2/afe/sv_pwm ==
  duties_uvw : Inport
  Bus Selector2 : BusSelector  OutputSignals=du(k),dv(k),dw(k)
  Constant1 : Constant  Value=afe_pwm_phase_shift_mod2
  modulator1 : Subsystem
  td2tc_1 : TransferFcn  Denominator=[tc 1]
  td2tc_2 : TransferFcn  Denominator=[tc 1]
  td2tc_3 : TransferFcn  Denominator=[tc 1]
  gate_cmds : Outport
  wires:
  td2tc_2/1 -> modulator1/2(v)  "dv(t)"
  td2tc_3/1 -> modulator1/3(w)  "dw(t)"
  td2tc_1/1 -> modulator1/1(u)  "du(t)"
  duties_uvw/1 -> Bus Selector2/1
  Bus Selector2/3 -> td2tc_3/1  "<dw(k)>"
  Bus Selector2/2 -> td2tc_2/1  "<dv(k)>"
  Bus Selector2/1 -> td2tc_1/1  "<du(k)>"
  Constant1/1 -> modulator1/4(phase)
  modulator1/1(gate_cmds) -> gate_cmds/1

== system afe_abc_inv_psm_n/afe_abc_inv_psm_mod2/afe/switch_1 ==
  Diode : fl_lib/Electrical/Electrical Elements/Diode  Vf=Vgamma V  Ron=Ron Ohm  Goff=1e-8 1/Ohm  i_specify=off  i_priority=None  i=0 A  i_nominal_specify=off  i_nominal_value=1  i_nominal_unit=A  v_specify=off  v_priority=None  v=0 V  v_nominal_specify=off  v_nominal_value=1  v_nominal_unit=V
  Switch : fl_lib/Electrical/Electrical Elements/Switch  R_closed=Ron Ohm  G_open=1e-8 1/Ohm  Threshold=7.5  i_specify=off  i_priority=None  i=0 A  i_nominal_specify=off  i_nominal_value=1  i_nominal_unit=A  v_specify=off  v_priority=None  v=0 V  v_nominal_specify=off  v_nominal_value=1  v_nominal_unit=V
  snubber : fl_lib/Electrical/Electrical Elements/Capacitor  c=Csnubber F  r=Rsnubber Ohm  g=0 1/Ohm  i_specify=off  i_priority=None  i=0 A  i_nominal_specify=off  i_nominal_value=1  i_nominal_unit=A  v_specify=off  v_priority=None  v=0 V  v_nominal_specify=off  v_nominal_value=1  v_nominal_unit=V  vc_specify=off  vc_priority=High  vc=0 V  vc_nominal_specify=off  vc_nominal_value=1  vc_nominal_unit=V
  G : PMIOPort  Side=Left
  C : PMIOPort  Port=2  Side=Left
  E : PMIOPort  Port=3  Side=Right
  connections:
  Switch/RConn2 -- C/RConn1 -- Diode/RConn1 -- snubber/LConn1
  Switch/RConn1 -- G/RConn1
  Switch/LConn1 -- E/RConn1 -- snubber/RConn1 -- Diode/LConn1

== system afe_abc_inv_psm_n/afe_abc_inv_psm_mod2/afe/switch_2 ==
  Diode : fl_lib/Electrical/Electrical Elements/Diode  Vf=Vgamma V  Ron=Ron Ohm  Goff=1e-8 1/Ohm  i_specify=off  i_priority=None  i=0 A  i_nominal_specify=off  i_nominal_value=1  i_nominal_unit=A  v_specify=off  v_priority=None  v=0 V  v_nominal_specify=off  v_nominal_value=1  v_nominal_unit=V
  Switch : fl_lib/Electrical/Electrical Elements/Switch  R_closed=Ron Ohm  G_open=1e-8 1/Ohm  Threshold=7.5  i_specify=off  i_priority=None  i=0 A  i_nominal_specify=off  i_nominal_value=1  i_nominal_unit=A  v_specify=off  v_priority=None  v=0 V  v_nominal_specify=off  v_nominal_value=1  v_nominal_unit=V
  snubber : fl_lib/Electrical/Electrical Elements/Capacitor  c=Csnubber F  r=Rsnubber Ohm  g=0 1/Ohm  i_specify=off  i_priority=None  i=0 A  i_nominal_specify=off  i_nominal_value=1  i_nominal_unit=A  v_specify=off  v_priority=None  v=0 V  v_nominal_specify=off  v_nominal_value=1  v_nominal_unit=V  vc_specify=off  vc_priority=High  vc=0 V  vc_nominal_specify=off  vc_nominal_value=1  vc_nominal_unit=V
  G : PMIOPort  Side=Left
  C : PMIOPort  Port=2  Side=Left
  E : PMIOPort  Port=3  Side=Right
  connections:
  Diode/LConn1 -- snubber/RConn1 -- E/RConn1 -- Switch/LConn1
  Switch/RConn1 -- G/RConn1
  Diode/RConn1 -- snubber/LConn1 -- C/RConn1 -- Switch/RConn2

== system afe_abc_inv_psm_n/afe_abc_inv_psm_mod2/afe/switch_3 ==
  Diode : fl_lib/Electrical/Electrical Elements/Diode  Vf=Vgamma V  Ron=Ron Ohm  Goff=1e-8 1/Ohm  i_specify=off  i_priority=None  i=0 A  i_nominal_specify=off  i_nominal_value=1  i_nominal_unit=A  v_specify=off  v_priority=None  v=0 V  v_nominal_specify=off  v_nominal_value=1  v_nominal_unit=V
  Switch : fl_lib/Electrical/Electrical Elements/Switch  R_closed=Ron Ohm  G_open=1e-8 1/Ohm  Threshold=7.5  i_specify=off  i_priority=None  i=0 A  i_nominal_specify=off  i_nominal_value=1  i_nominal_unit=A  v_specify=off  v_priority=None  v=0 V  v_nominal_specify=off  v_nominal_value=1  v_nominal_unit=V
  snubber : fl_lib/Electrical/Electrical Elements/Capacitor  c=Csnubber F  r=Rsnubber Ohm  g=0 1/Ohm  i_specify=off  i_priority=None  i=0 A  i_nominal_specify=off  i_nominal_value=1  i_nominal_unit=A  v_specify=off  v_priority=None  v=0 V  v_nominal_specify=off  v_nominal_value=1  v_nominal_unit=V  vc_specify=off  vc_priority=High  vc=0 V  vc_nominal_specify=off  vc_nominal_value=1  vc_nominal_unit=V
  G : PMIOPort  Side=Left
  C : PMIOPort  Port=2  Side=Left
  E : PMIOPort  Port=3  Side=Right
  connections:
  Diode/LConn1 -- snubber/RConn1 -- E/RConn1 -- Switch/LConn1
  Switch/RConn1 -- G/RConn1
  Diode/RConn1 -- snubber/LConn1 -- C/RConn1 -- Switch/RConn2

== system afe_abc_inv_psm_n/afe_abc_inv_psm_mod2/afe/switch_4 ==
  Diode : fl_lib/Electrical/Electrical Elements/Diode  Vf=Vgamma V  Ron=Ron Ohm  Goff=1e-8 1/Ohm  i_specify=off  i_priority=None  i=0 A  i_nominal_specify=off  i_nominal_value=1  i_nominal_unit=A  v_specify=off  v_priority=None  v=0 V  v_nominal_specify=off  v_nominal_value=1  v_nominal_unit=V
  Switch : fl_lib/Electrical/Electrical Elements/Switch  R_closed=Ron Ohm  G_open=1e-8 1/Ohm  Threshold=7.5  i_specify=off  i_priority=None  i=0 A  i_nominal_specify=off  i_nominal_value=1  i_nominal_unit=A  v_specify=off  v_priority=None  v=0 V  v_nominal_specify=off  v_nominal_value=1  v_nominal_unit=V
  snubber : fl_lib/Electrical/Electrical Elements/Capacitor  c=Csnubber F  r=Rsnubber Ohm  g=0 1/Ohm  i_specify=off  i_priority=None  i=0 A  i_nominal_specify=off  i_nominal_value=1  i_nominal_unit=A  v_specify=off  v_priority=None  v=0 V  v_nominal_specify=off  v_nominal_value=1  v_nominal_unit=V  vc_specify=off  vc_priority=High  vc=0 V  vc_nominal_specify=off  vc_nominal_value=1  vc_nominal_unit=V
  G : PMIOPort  Side=Left
  C : PMIOPort  Port=2  Side=Left
  E : PMIOPort  Port=3  Side=Right
  connections:
  Diode/RConn1 -- snubber/LConn1 -- Switch/RConn2 -- C/RConn1
  Switch/RConn1 -- G/RConn1
  Diode/LConn1 -- snubber/RConn1 -- Switch/LConn1 -- E/RConn1
